simulink model "beaglebone_logi"  (R2014b)
settings: Solver=FixedStepDiscrete  StartTime=0.0  StopTime=inf  RelTol=1e-3
settings Model: ModifiedByFormat=The MathWorks Inc.  SimulationMode=external  Creator=The MathWorks Inc.  LastModifiedBy=The MathWorks Inc.
settings OptimizationCC: OptimizeModelRefInitCode=on  LifeSpan=Inf  MaxStackSize=64
settings DebuggingCC: UnderspecifiedInitializationDetection=Classic  MergeDetectMultiDrivingBlocksExec=none
settings HardwareCC: ProdLargestAtomicInteger=Long  ProdLargestAtomicFloat=Double  ProdEndianess=LittleEndian  ProdHWDeviceType=ARM Compatible->ARM Cortex
settings RTWCC: SystemTargetFile=ert.tlc  TemplateMakefile=ert_default_tmf  Description=Embedded Coder  ProcessScript=ert_make_rtw_hook  Toolchain=Linaro Toolchain v4.8
settings CodeAppCC: IgnoreCustomStorageClasses=off
settings ERTTargetCC: ExtMode=on  ExtModeMexArgs='10.10.10.133'

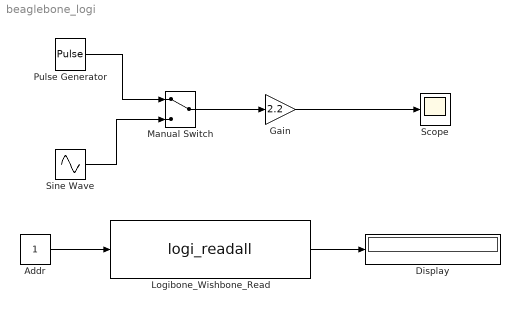
== system beaglebone_logi ==
  Addr : Constant  OutDataTypeStr=Inherit: Inherit via back propagation
  Display : Display
      settings: Format=hex (Stored Integer)
  Gain : Gain  Gain=2.2
  Logibone_Wishbone_Read : S-Function  InitFcn=try, set_param(gcb,'FunctionName','logi_readall'), end  FunctionName=logi_readall  SFunctionModules=logi_readall_wrapper  EnableBusSupport=off  mask(S-Function Builder){}
      mask help: Simulink:masks:SFunctionBuilder_MD
      mask init:
      | val = [[.9  0.75 0.75 1 1 .9 .9 1]',[1 1 0.75 0.75 .9 .9 1 .9]'];try , sys = get_param(gcb,'SfunBuilderFcnName');if isempty(sys), sys = get_param(gcb,'FunctionName'); end,catch, sys = get_param(gcb,'FunctionName'); end
      settings: CopyFcn=set_param(gcbh,'LinkStatus','none')  PreSaveFcn=try, set_param(gcb,'FunctionName','logi_readall'), end  OpenFcn=sfunctionwizard(gcbh)
      mask Display: plot(val(:,1),val(:,2)),disp(sys), port_label('input',1,'address'), port_label('output',1,'data')
  Manual Switch : ManualSwitch
  Pulse Generator : DiscretePulseGenerator  Period=10  PulseWidth=5  SampleTime=0.1
  Scope : Scope
      settings: TimeRange=10  YMin=0
  Sine Wave : Sin  SineType=Sample based  SampleTime=0.1
  wires:
  Manual Switch/1 -> Gain/1
  Gain/1 -> Scope/1
  Pulse Generator/1 -> Manual Switch/1
  Sine Wave/1 -> Manual Switch/2
  Addr/1 -> Logibone_Wishbone_Read/1
  Logibone_Wishbone_Read/1 -> Display/1
